simulink model "ProyectoFinal"  (R2018b)
settings: Solver=VariableStepAuto  StartTime=0.0  StopTime=100  RelTol=1e-3
libraries: simulink x3
settings Model: Creator=alvar  LastModifiedBy=alvar

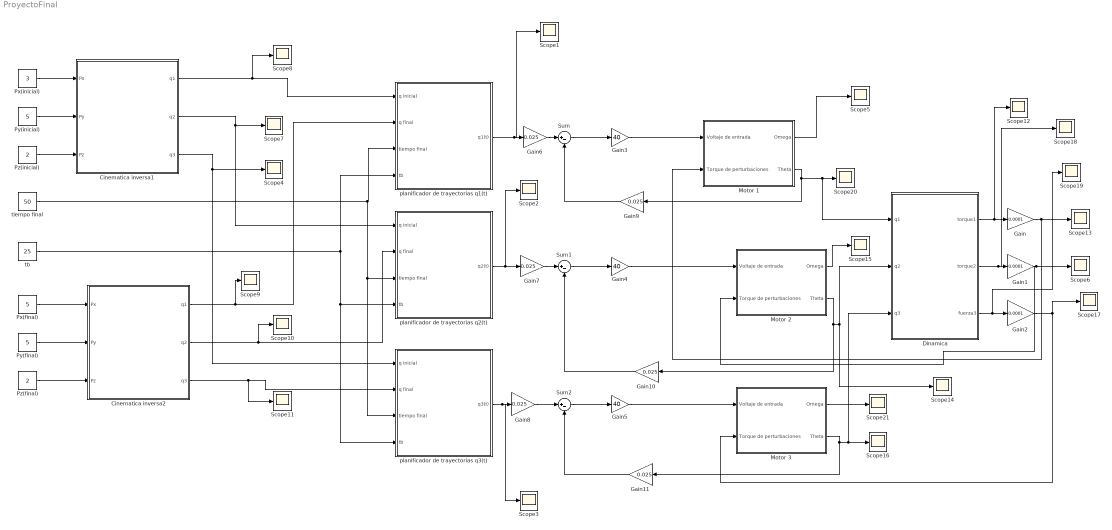
== system ProyectoFinal ==
  Cinematica inversa1 : Subsystem
  Cinematica inversa2 : Subsystem
  Dinamica : Subsystem
  Gain : Gain  Gain=0.0001
  Gain1 : Gain  Gain=0.0001
  Gain{6..11} (6 alike) : Gain  Gain=0.025
  Gain2 : Gain  Gain=0.0001
  Gain3 : Gain  Gain=40
  Gain4 : Gain  Gain=40
  Gain5 : Gain  Gain=40
  "Motor 1 " : Subsystem
  "Motor 2 " : Subsystem
  Motor 3 : Subsystem
  Px(final) : Constant  Value=5
  Px(inicial) : Constant  Value=3
  Py(final) : Constant  Value=5
  Py(inicial) : Constant  Value=5
  Pz(final) : Constant  Value=2
  Pz(inicial) : Constant  Value=2
  Scope{1..21} (21 alike) : Scope
  Sum : Sum  Inputs=|+-
  Sum1 : Sum  Inputs=|+-
  Sum2 : Sum  Inputs=|+-
  planificador de trayectorias q1(t) : Subsystem
  planificador de trayectorias q2(t) : Subsystem
  planificador de trayectorias q3(t) : Subsystem
  tb : Constant  Value=25
  tiempo final : Constant  Value=50
  wires:
  Motor 3/1(Omega) -> Scope21/1
  Gain11/1 -> Sum2/2
  Gain10/1 -> Sum1/2
  Gain9/1 -> Sum/2
  Sum/1 -> Gain3/1
  Sum2/1 -> Gain5/1
  Pz(inicial)/1 -> Cinematica inversa1/3(Pz)
  Px(inicial)/1 -> Cinematica inversa1/1(Px)
  Cinematica inversa2/1(q1) -> Scope9/1, planificador de trayectorias q1(t)/2(q final)
  Cinematica inversa1/1(q1) -> Scope8/1, planificador de trayectorias q1(t)/1(q inicial)
  Cinematica inversa1/2(q2) -> Scope7/1, planificador de trayectorias q2(t)/1(q inicial)
  Cinematica inversa2/3(q3) -> Scope11/1, planificador de trayectorias q3(t)/2(q final)
  tb/1 -> planificador de trayectorias q3(t)/4(tb), planificador de trayectorias q2(t)/4(tb), planificador de trayectorias q1(t)/4(tb)
  Gain5/1 -> Motor 3/1(Voltaje de entrada)
  Py(final)/1 -> Cinematica inversa2/2(Py)
  Py(inicial)/1 -> Cinematica inversa1/2(Py)
  Pz(final)/1 -> Cinematica inversa2/3(Pz)
  tiempo final/1 -> planificador de trayectorias q3(t)/3(tiempo final), planificador de trayectorias q2(t)/3(tiempo final), planificador de trayectorias q1(t)/3(tiempo final)
  planificador de trayectorias q2(t)/1("q2(t) ") -> Gain7/1, Scope2/1
  Px(final)/1 -> Cinematica inversa2/1(Px)
  Gain7/1 -> Sum1/1
  Gain3/1 -> "Motor 1 "/1(Voltaje de entrada)
  planificador de trayectorias q3(t)/1("q3(t) ") -> Scope3/1, Gain8/1
  Gain1/1 -> "Motor 2 "/2(Torque de perturbaciones), Scope6/1
  Dinamica/3(fuerza3) -> Scope19/1, Gain2/1
  Cinematica inversa2/2(q2) -> Scope10/1, planificador de trayectorias q2(t)/2(q final)
  planificador de trayectorias q1(t)/1("q1(t) ") -> Scope1/1, Gain6/1
  Dinamica/1(torque1) -> Scope12/1, Gain/1
  Dinamica/2(torque2) -> Scope18/1, Gain1/1
  Gain2/1 -> Motor 3/2(Torque de perturbaciones), Scope17/1
  Gain6/1 -> Sum/1
  Gain/1 -> Scope13/1, "Motor 1 "/2(Torque de perturbaciones)
  Motor 3/2(Theta) -> Gain11/1, Scope16/1, Dinamica/3(q3)
  "Motor 1 "/2(Theta) -> Dinamica/1(q1), Scope20/1, Gain9/1
  "Motor 2 "/1(Omega) -> Scope15/1
  "Motor 2 "/2(Theta) -> Scope14/1, Dinamica/2(q2), Gain10/1
  Sum1/1 -> Gain4/1
  Gain8/1 -> Sum2/1
  Cinematica inversa1/3(q3) -> Scope4/1, planificador de trayectorias q3(t)/1(q inicial)
  "Motor 1 "/1(Omega) -> Scope5/1
  Gain4/1 -> "Motor 2 "/1(Voltaje de entrada)

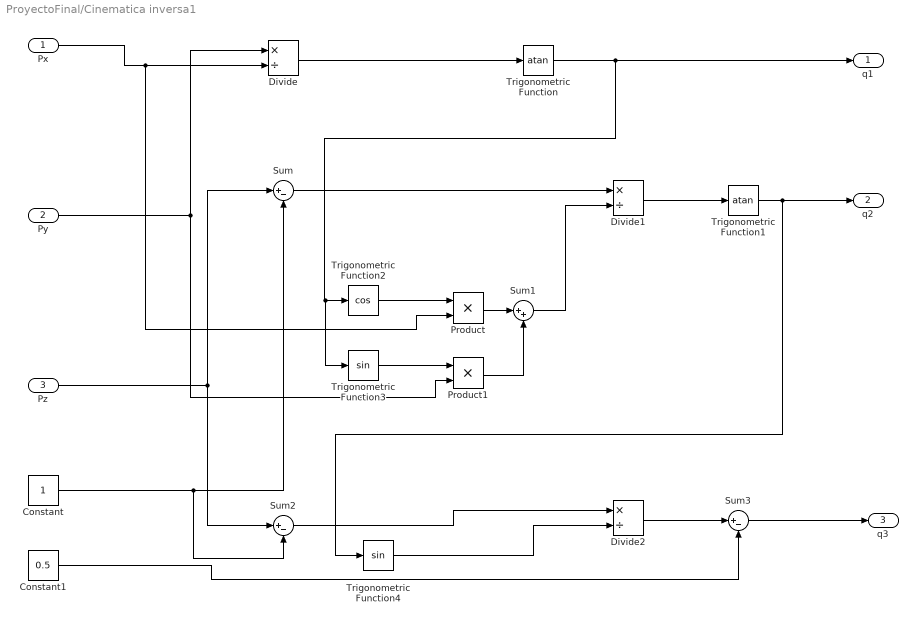
== system ProyectoFinal/Cinematica inversa1 ==
  Px : Inport
  Py : Inport  Port=2
  Pz : Inport  Port=3
  Constant : Constant
  Constant1 : Constant  Value=0.5
  Divide : Product  Inputs=*/
  Divide1 : Product  Inputs=*/
  Divide2 : Product  Inputs=*/
  Product : Product
  Product1 : Product
  Sum : Sum  Inputs=|+-
  Sum1 : Sum  Inputs=|++
  Sum2 : Sum  Inputs=|+-
  Sum3 : Sum  Inputs=|+-
  Trigonometric Function : Trigonometry  Operator=atan
  Trigonometric Function1 : Trigonometry  Operator=atan
  Trigonometric Function2 : Trigonometry  Operator=cos
  Trigonometric Function3 : Trigonometry
  Trigonometric Function4 : Trigonometry
  q1 : Outport
  q2 : Outport  Port=2
  q3 : Outport  Port=3
  wires:
  Py/1 -> Product1/2, Divide/1
  Px/1 -> Product/2, Divide/2
  Divide/1 -> Trigonometric Function/1
  Trigonometric Function/1 -> Trigonometric Function3/1, Trigonometric Function2/1, q1/1
  Pz/1 -> Sum/1, Sum2/1
  Constant/1 -> Sum2/2, Sum/2
  Sum/1 -> Divide1/1
  Trigonometric Function2/1 -> Product/1
  Product/1 -> Sum1/1
  Trigonometric Function3/1 -> Product1/1
  Product1/1 -> Sum1/2
  Sum1/1 -> Divide1/2
  Divide1/1 -> Trigonometric Function1/1
  Trigonometric Function1/1 -> Trigonometric Function4/1, q2/1
  Sum2/1 -> Divide2/1
  Trigonometric Function4/1 -> Divide2/2
  Divide2/1 -> Sum3/1
  Sum3/1 -> q3/1
  Constant1/1 -> Sum3/2

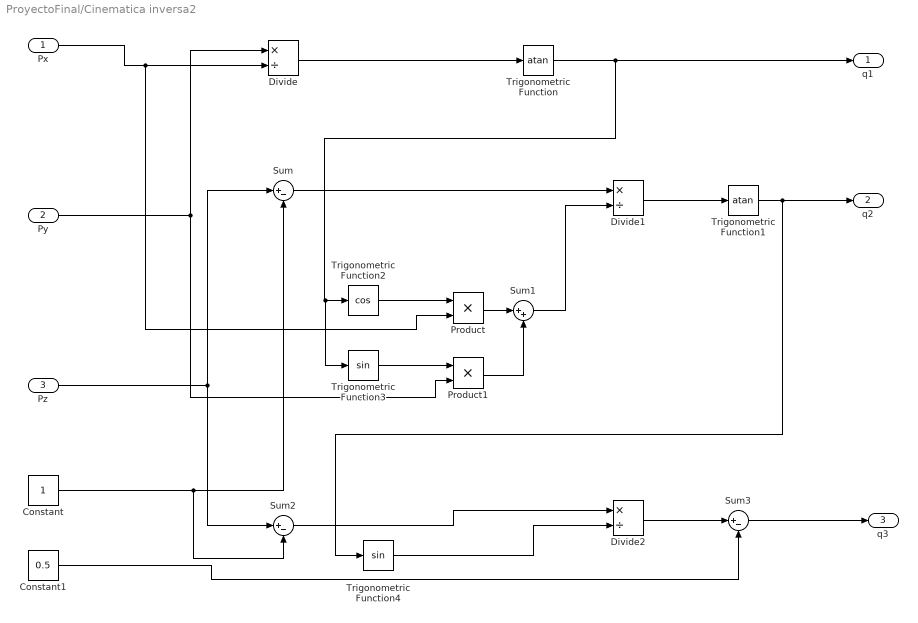
== system ProyectoFinal/Cinematica inversa2 ==
  Px : Inport
  Py : Inport  Port=2
  Pz : Inport  Port=3
  Constant : Constant
  Constant1 : Constant  Value=0.5
  Divide : Product  Inputs=*/
  Divide1 : Product  Inputs=*/
  Divide2 : Product  Inputs=*/
  Product : Product
  Product1 : Product
  Sum : Sum  Inputs=|+-
  Sum1 : Sum  Inputs=|++
  Sum2 : Sum  Inputs=|+-
  Sum3 : Sum  Inputs=|+-
  Trigonometric Function : Trigonometry  Operator=atan
  Trigonometric Function1 : Trigonometry  Operator=atan
  Trigonometric Function2 : Trigonometry  Operator=cos
  Trigonometric Function3 : Trigonometry
  Trigonometric Function4 : Trigonometry
  q1 : Outport
  q2 : Outport  Port=2
  q3 : Outport  Port=3
  wires:
  Py/1 -> Product1/2, Divide/1
  Px/1 -> Product/2, Divide/2
  Divide/1 -> Trigonometric Function/1
  Trigonometric Function/1 -> Trigonometric Function3/1, Trigonometric Function2/1, q1/1
  Pz/1 -> Sum/1, Sum2/1
  Constant/1 -> Sum2/2, Sum/2
  Sum/1 -> Divide1/1
  Trigonometric Function2/1 -> Product/1
  Product/1 -> Sum1/1
  Trigonometric Function3/1 -> Product1/1
  Product1/1 -> Sum1/2
  Sum1/1 -> Divide1/2
  Divide1/1 -> Trigonometric Function1/1
  Trigonometric Function1/1 -> Trigonometric Function4/1, q2/1
  Sum2/1 -> Divide2/1
  Trigonometric Function4/1 -> Divide2/2
  Divide2/1 -> Sum3/1
  Sum3/1 -> q3/1
  Constant1/1 -> Sum3/2

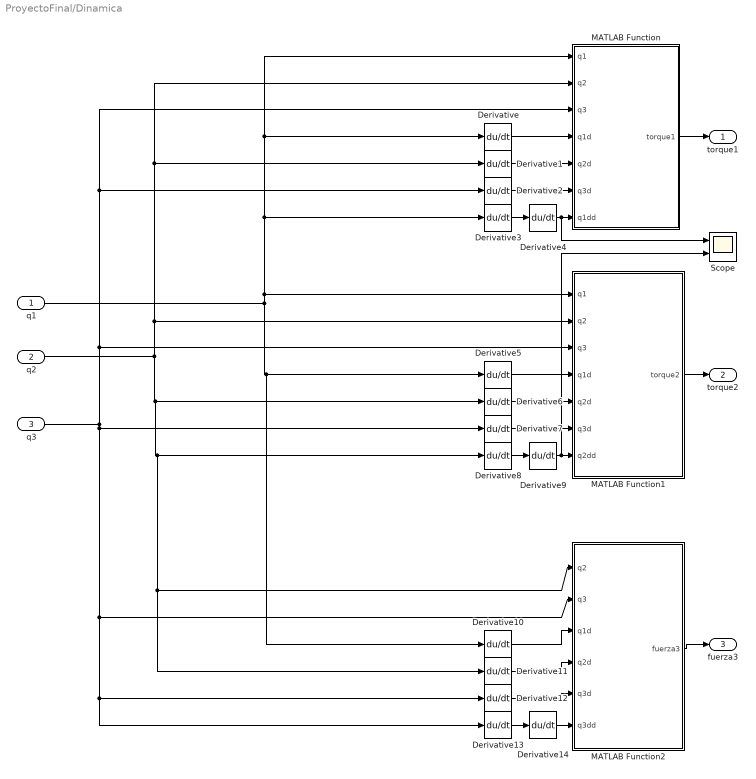
== system ProyectoFinal/Dinamica ==
  q1 : Inport
  q2 : Inport  Port=2
  q3 : Inport  Port=3
  Derivative{,1..14} (15 alike) : Derivative
  MATLAB Function : MATLAB Function  TreatAsAtomicUnit=on
  MATLAB Function1 : MATLAB Function  TreatAsAtomicUnit=on
  MATLAB Function2 : MATLAB Function  TreatAsAtomicUnit=on
  Scope : Scope  NumInputPorts=2
  torque1 : Outport
  torque2 : Outport  Port=2
  fuerza3 : Outport  Port=3
  wires:
  Derivative5/1 -> MATLAB Function1/4(q1d)
  MATLAB Function1/1(torque2) -> torque2/1
  Derivative4/1 -> Scope/1, MATLAB Function/7(q1dd)
  Derivative3/1 -> Derivative4/1
  Derivative14/1 -> MATLAB Function2/6(q3dd)
  Derivative7/1 -> MATLAB Function1/6(q3d)
  q1/1 -> Derivative10/1, Derivative5/1, MATLAB Function1/1(q1), Derivative3/1, Derivative/1, MATLAB Function/1(q1)
  Derivative6/1 -> MATLAB Function1/5(q2d)
  Derivative8/1 -> Derivative9/1
  Derivative9/1 -> Scope/2, MATLAB Function1/7(q2dd)
  Derivative1/1 -> MATLAB Function/5(q2d)
  Derivative/1 -> MATLAB Function/4(q1d)
  Derivative2/1 -> MATLAB Function/6(q3d)
  MATLAB Function2/1(fuerza3) -> fuerza3/1
  Derivative11/1 -> MATLAB Function2/4(q2d)
  Derivative13/1 -> Derivative14/1
  Derivative12/1 -> MATLAB Function2/5(q3d)
  Derivative10/1 -> MATLAB Function2/3(q1d)
  q2/1 -> MATLAB Function2/1(q2), Derivative11/1, Derivative8/1, Derivative6/1, MATLAB Function1/2(q2), Derivative1/1, MATLAB Function/2(q2)
  q3/1 -> Derivative13/1, Derivative12/1, MATLAB Function2/2(q3), Derivative7/1, MATLAB Function1/3(q3), Derivative2/1, MATLAB Function/3(q3)
  MATLAB Function/1(torque1) -> torque1/1

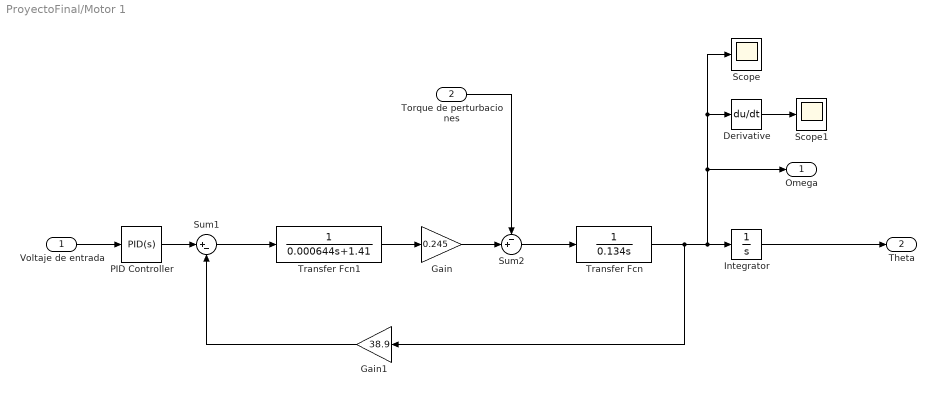
== system ProyectoFinal/Motor 1  ==
  Voltaje de entrada : Inport
  Torque de perturbaciones : Inport  Port=2
  Derivative : Derivative
  Gain : Gain  Gain=0.245
  Gain1 : Gain  Gain=38.9
  Integrator : Integrator
  PID Controller : simulink/Continuous/PID Controller  Controller=PID  Form=Parallel  TimeDomain=Continuous-time  SampleTime=-1  IntegratorMethod=Forward Euler  FilterMethod=Forward Euler  ControllerParametersSource=internal  P=12  I=4  D=5  UseFilter=on  N=100  TunerSelectOption=Transfer Function Based (PID Tuner App)  InitialConditionSource=internal  InitialConditionForIntegrator=0  InitialConditionForFilter=0  DifferentiatorICPrevScaledInput=0  ExternalReset=none  TrackingMode=off  Kt=1  LimitOutput=off  UpperSaturationLimit=inf  LowerSaturationLimit=-inf  LinearizeAsGain=on  AntiWindupMode=none  Kb=1  POutMin=[]  POutMax=[]  IOutMin=[]  IOutMax=[]  DOutMin=[]  DOutMax=[]  NOutMin=[]  NOutMax=[]  SumOutMin=[]  SumOutMax=[]  SaturationOutMin=[]  SaturationOutMax=[]  PParamMin=[]  PParamMax=[]  IParamMin=[]  IParamMax=[]  DParamMin=[]  DParamMax=[]  NParamMin=[]  NParamMax=[]  KbParamMin=[]  KbParamMax=[]  KtParamMin=[]  KtParamMax=[]  KbOutMin=[]  KbOutMax=[]  KtOutMin=[]  KtOutMax=[]  IntegratorOutMin=[]  IntegratorOutMax=[]  FilterOutMin=[]  FilterOutMax=[]  SumI1OutMin=[]  SumI1OutMax=[]  SumI2OutMin=[]  SumI2OutMax=[]  SumI3OutMin=[]  SumI3OutMax=[]  SumI4OutMin=[]  SumI4OutMax=[]  SumDOutMin=[]  SumDOutMax=[]  DifferentiatorOutMin=[]  DifferentiatorOutMax=[]  FilterDiffOutCoefMin=[]  FilterDiffOutCoefMax=[]  ReciprocalOutMin=[]  ReciprocalOutMax=[]  SumDenOutMin=[]  SumDenOutMax=[]  SumNumOutMin=[]  SumNumOutMax=[]  DivideOutMin=[]  DivideOutMax=[]  IntegratorContinuousStateAttributes=''  IntegratorStateMustResolveToSignalObject=off  IntegratorRTWStateStorageClass=Auto  FilterContinuousStateAttributes=''  FilterStateMustResolveToSignalObject=off  FilterRTWStateStorageClass=Auto  ParallelPVariant=InternalParameters  IdealPVariant=Disabled  IVariant=InternalParameters  DVariant=InternalParameters  IntegratorVariant=Continuous  SatVariant=Disabled  AWVariant=Passthrough  PCopyVariant=Disabled  TRVariant=Disabled  FdbkBlocksVariant=Forward  IdealPFdbkVariant=Disabled  SatFdbkVariant=Disabled  DerivativeFilterVariant=ContFilter  NVariant=InternalParameters  NCopyVariant=Disabled  FilterICVariant=InternalICsFilter  IntegratorICVariant=InternalICs  ExternalResetVariant=Disabled  TRSumVariant=Passthrough  SumFdbkVariant=Disabled  SumVariant=Sum_PID
  Scope : Scope
  Scope1 : Scope
  Sum1 : Sum  Inputs=|+-
  Sum2 : Sum  Inputs=-+|
  Transfer Fcn : TransferFcn  Denominator=[0.134 0]
  Transfer Fcn1 : TransferFcn  Denominator=[0.000644 1.41]
  Omega : Outport
  Theta : Outport  Port=2
  wires:
  Sum1/1 -> Transfer Fcn1/1
  Transfer Fcn1/1 -> Gain/1
  Gain1/1 -> Sum1/2
  Gain/1 -> Sum2/2
  Sum2/1 -> Transfer Fcn/1
  Torque de perturbaciones/1 -> Sum2/1
  Integrator/1 -> Theta/1
  Derivative/1 -> Scope1/1
  Transfer Fcn/1 -> Derivative/1, Scope/1, Omega/1, Integrator/1, Gain1/1
  PID Controller/1 -> Sum1/1
  Voltaje de entrada/1 -> PID Controller/1

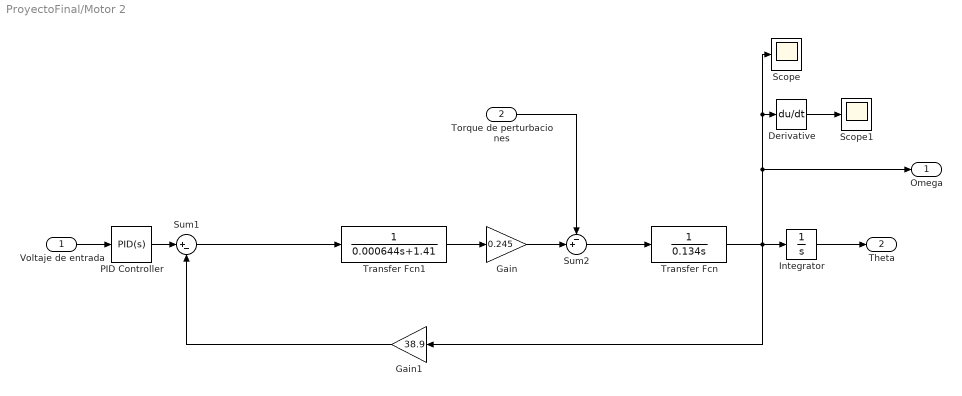
== system ProyectoFinal/Motor 2  ==
  Voltaje de entrada : Inport
  Torque de perturbaciones : Inport  Port=2
  Derivative : Derivative
  Gain : Gain  Gain=0.245
  Gain1 : Gain  Gain=38.9
  Integrator : Integrator
  PID Controller : simulink/Continuous/PID Controller  Controller=PID  Form=Parallel  TimeDomain=Continuous-time  SampleTime=-1  IntegratorMethod=Forward Euler  FilterMethod=Forward Euler  ControllerParametersSource=internal  P=12  I=4  D=5  UseFilter=on  N=100  TunerSelectOption=Transfer Function Based (PID Tuner App)  InitialConditionSource=internal  InitialConditionForIntegrator=0  InitialConditionForFilter=0  DifferentiatorICPrevScaledInput=0  ExternalReset=none  TrackingMode=off  Kt=1  LimitOutput=off  UpperSaturationLimit=inf  LowerSaturationLimit=-inf  LinearizeAsGain=on  AntiWindupMode=none  Kb=1  POutMin=[]  POutMax=[]  IOutMin=[]  IOutMax=[]  DOutMin=[]  DOutMax=[]  NOutMin=[]  NOutMax=[]  SumOutMin=[]  SumOutMax=[]  SaturationOutMin=[]  SaturationOutMax=[]  PParamMin=[]  PParamMax=[]  IParamMin=[]  IParamMax=[]  DParamMin=[]  DParamMax=[]  NParamMin=[]  NParamMax=[]  KbParamMin=[]  KbParamMax=[]  KtParamMin=[]  KtParamMax=[]  KbOutMin=[]  KbOutMax=[]  KtOutMin=[]  KtOutMax=[]  IntegratorOutMin=[]  IntegratorOutMax=[]  FilterOutMin=[]  FilterOutMax=[]  SumI1OutMin=[]  SumI1OutMax=[]  SumI2OutMin=[]  SumI2OutMax=[]  SumI3OutMin=[]  SumI3OutMax=[]  SumI4OutMin=[]  SumI4OutMax=[]  SumDOutMin=[]  SumDOutMax=[]  DifferentiatorOutMin=[]  DifferentiatorOutMax=[]  FilterDiffOutCoefMin=[]  FilterDiffOutCoefMax=[]  ReciprocalOutMin=[]  ReciprocalOutMax=[]  SumDenOutMin=[]  SumDenOutMax=[]  SumNumOutMin=[]  SumNumOutMax=[]  DivideOutMin=[]  DivideOutMax=[]  IntegratorContinuousStateAttributes=''  IntegratorStateMustResolveToSignalObject=off  IntegratorRTWStateStorageClass=Auto  FilterContinuousStateAttributes=''  FilterStateMustResolveToSignalObject=off  FilterRTWStateStorageClass=Auto  ParallelPVariant=InternalParameters  IdealPVariant=Disabled  IVariant=InternalParameters  DVariant=InternalParameters  IntegratorVariant=Continuous  SatVariant=Disabled  AWVariant=Passthrough  PCopyVariant=Disabled  TRVariant=Disabled  FdbkBlocksVariant=Forward  IdealPFdbkVariant=Disabled  SatFdbkVariant=Disabled  DerivativeFilterVariant=ContFilter  NVariant=InternalParameters  NCopyVariant=Disabled  FilterICVariant=InternalICsFilter  IntegratorICVariant=InternalICs  ExternalResetVariant=Disabled  TRSumVariant=Passthrough  SumFdbkVariant=Disabled  SumVariant=Sum_PID
  Scope : Scope
  Scope1 : Scope
  Sum1 : Sum  Inputs=|+-
  Sum2 : Sum  Inputs=-+|
  Transfer Fcn : TransferFcn  Denominator=[0.134 0]
  Transfer Fcn1 : TransferFcn  Denominator=[0.000644 1.41]
  Omega : Outport
  Theta : Outport  Port=2
  wires:
  Sum1/1 -> Transfer Fcn1/1
  Transfer Fcn1/1 -> Gain/1
  Gain1/1 -> Sum1/2
  Gain/1 -> Sum2/2
  Sum2/1 -> Transfer Fcn/1
  Torque de perturbaciones/1 -> Sum2/1
  Integrator/1 -> Theta/1
  Derivative/1 -> Scope1/1
  Transfer Fcn/1 -> Gain1/1, Omega/1, Derivative/1, Scope/1, Integrator/1
  PID Controller/1 -> Sum1/1
  Voltaje de entrada/1 -> PID Controller/1

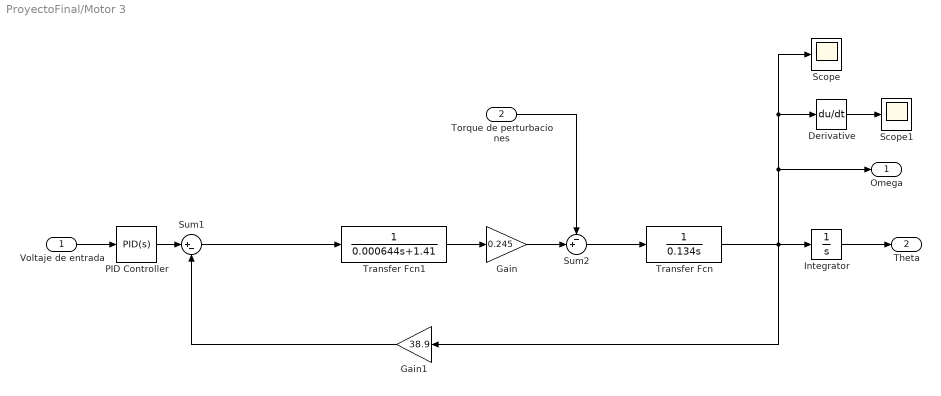
== system ProyectoFinal/Motor 3 ==
  Voltaje de entrada : Inport
  Torque de perturbaciones : Inport  Port=2
  Derivative : Derivative
  Gain : Gain  Gain=0.245
  Gain1 : Gain  Gain=38.9
  Integrator : Integrator
  PID Controller : simulink/Continuous/PID Controller  Controller=PID  Form=Parallel  TimeDomain=Continuous-time  SampleTime=-1  IntegratorMethod=Forward Euler  FilterMethod=Forward Euler  ControllerParametersSource=internal  P=12  I=4  D=5  UseFilter=on  N=100  TunerSelectOption=Transfer Function Based (PID Tuner App)  InitialConditionSource=internal  InitialConditionForIntegrator=0  InitialConditionForFilter=0  DifferentiatorICPrevScaledInput=0  ExternalReset=none  TrackingMode=off  Kt=1  LimitOutput=off  UpperSaturationLimit=inf  LowerSaturationLimit=-inf  LinearizeAsGain=on  AntiWindupMode=none  Kb=1  POutMin=[]  POutMax=[]  IOutMin=[]  IOutMax=[]  DOutMin=[]  DOutMax=[]  NOutMin=[]  NOutMax=[]  SumOutMin=[]  SumOutMax=[]  SaturationOutMin=[]  SaturationOutMax=[]  PParamMin=[]  PParamMax=[]  IParamMin=[]  IParamMax=[]  DParamMin=[]  DParamMax=[]  NParamMin=[]  NParamMax=[]  KbParamMin=[]  KbParamMax=[]  KtParamMin=[]  KtParamMax=[]  KbOutMin=[]  KbOutMax=[]  KtOutMin=[]  KtOutMax=[]  IntegratorOutMin=[]  IntegratorOutMax=[]  FilterOutMin=[]  FilterOutMax=[]  SumI1OutMin=[]  SumI1OutMax=[]  SumI2OutMin=[]  SumI2OutMax=[]  SumI3OutMin=[]  SumI3OutMax=[]  SumI4OutMin=[]  SumI4OutMax=[]  SumDOutMin=[]  SumDOutMax=[]  DifferentiatorOutMin=[]  DifferentiatorOutMax=[]  FilterDiffOutCoefMin=[]  FilterDiffOutCoefMax=[]  ReciprocalOutMin=[]  ReciprocalOutMax=[]  SumDenOutMin=[]  SumDenOutMax=[]  SumNumOutMin=[]  SumNumOutMax=[]  DivideOutMin=[]  DivideOutMax=[]  IntegratorContinuousStateAttributes=''  IntegratorStateMustResolveToSignalObject=off  IntegratorRTWStateStorageClass=Auto  FilterContinuousStateAttributes=''  FilterStateMustResolveToSignalObject=off  FilterRTWStateStorageClass=Auto  ParallelPVariant=InternalParameters  IdealPVariant=Disabled  IVariant=InternalParameters  DVariant=InternalParameters  IntegratorVariant=Continuous  SatVariant=Disabled  AWVariant=Passthrough  PCopyVariant=Disabled  TRVariant=Disabled  FdbkBlocksVariant=Forward  IdealPFdbkVariant=Disabled  SatFdbkVariant=Disabled  DerivativeFilterVariant=ContFilter  NVariant=InternalParameters  NCopyVariant=Disabled  FilterICVariant=InternalICsFilter  IntegratorICVariant=InternalICs  ExternalResetVariant=Disabled  TRSumVariant=Passthrough  SumFdbkVariant=Disabled  SumVariant=Sum_PID
  Scope : Scope
  Scope1 : Scope
  Sum1 : Sum  Inputs=|+-
  Sum2 : Sum  Inputs=-+|
  Transfer Fcn : TransferFcn  Denominator=[0.134 0]
  Transfer Fcn1 : TransferFcn  Denominator=[0.000644 1.41]
  Omega : Outport
  Theta : Outport  Port=2
  wires:
  Sum1/1 -> Transfer Fcn1/1
  Transfer Fcn1/1 -> Gain/1
  Gain1/1 -> Sum1/2
  Gain/1 -> Sum2/2
  Sum2/1 -> Transfer Fcn/1
  Torque de perturbaciones/1 -> Sum2/1
  Integrator/1 -> Theta/1
  Derivative/1 -> Scope1/1
  Transfer Fcn/1 -> Omega/1, Derivative/1, Scope/1, Integrator/1, Gain1/1
  PID Controller/1 -> Sum1/1
  Voltaje de entrada/1 -> PID Controller/1

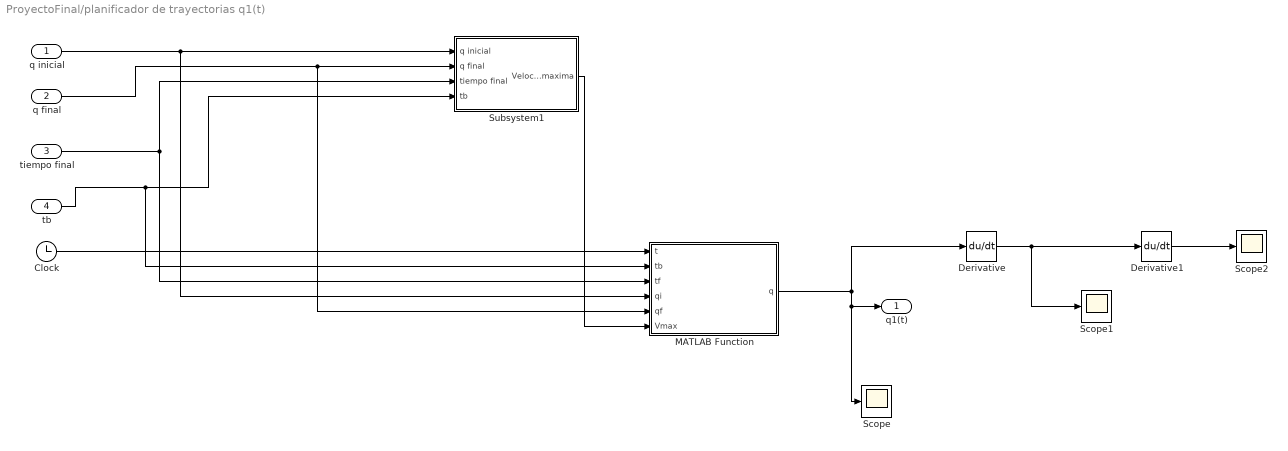
== system ProyectoFinal/planificador de trayectorias q1(t) ==
  q inicial : Inport
  q final : Inport  Port=2
  tiempo final : Inport  Port=3
  tb : Inport  Port=4
  Clock : Clock
  Derivative : Derivative
  Derivative1 : Derivative
  MATLAB Function : MATLAB Function  TreatAsAtomicUnit=on
  Scope : Scope
  Scope1 : Scope
  Scope2 : Scope
  Subsystem1 : Subsystem
  "q1(t) " : Outport
  wires:
  tb/1 -> Subsystem1/4(tb), MATLAB Function/2(tb)
  q final/1 -> MATLAB Function/5(qf), Subsystem1/2(q final)
  Derivative1/1 -> Scope2/1
  Derivative/1 -> Scope1/1, Derivative1/1
  Subsystem1/1(Velocidad maxima) -> MATLAB Function/6(Vmax)
  Clock/1 -> MATLAB Function/1(t)
  q inicial/1 -> MATLAB Function/4(qi), Subsystem1/1(q inicial)
  tiempo final/1 -> MATLAB Function/3(tf), Subsystem1/3(tiempo final)
  MATLAB Function/1(q) -> Derivative/1, "q1(t) "/1, Scope/1

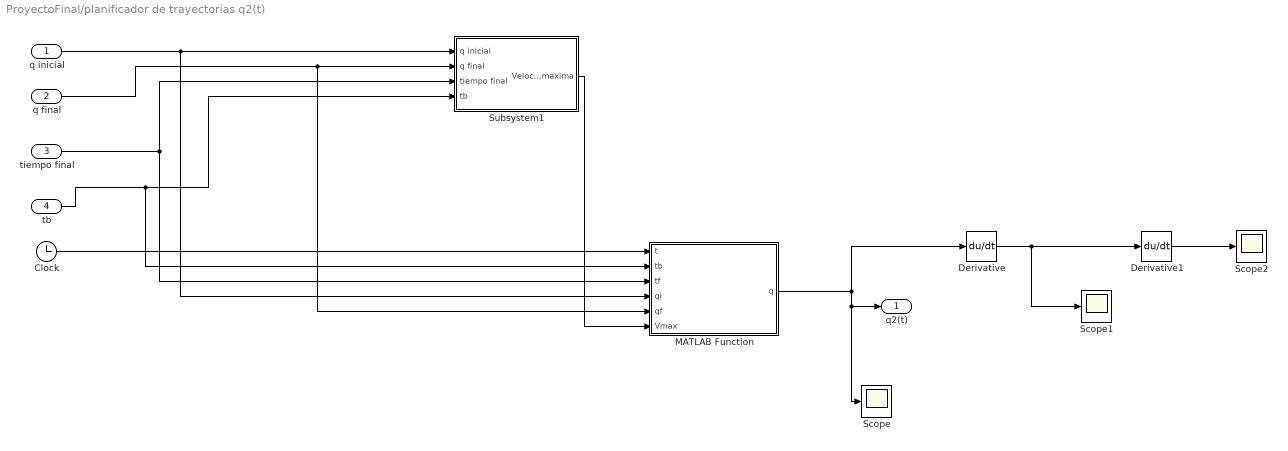
== system ProyectoFinal/planificador de trayectorias q2(t) ==
  q inicial : Inport
  q final : Inport  Port=2
  tiempo final : Inport  Port=3
  tb : Inport  Port=4
  Clock : Clock
  Derivative : Derivative
  Derivative1 : Derivative
  MATLAB Function : MATLAB Function  TreatAsAtomicUnit=on
  Scope : Scope
  Scope1 : Scope
  Scope2 : Scope
  Subsystem1 : Subsystem
  "q2(t) " : Outport
  wires:
  tb/1 -> Subsystem1/4(tb), MATLAB Function/2(tb)
  q final/1 -> MATLAB Function/5(qf), Subsystem1/2(q final)
  Derivative1/1 -> Scope2/1
  Derivative/1 -> Scope1/1, Derivative1/1
  Subsystem1/1(Velocidad maxima) -> MATLAB Function/6(Vmax)
  Clock/1 -> MATLAB Function/1(t)
  q inicial/1 -> MATLAB Function/4(qi), Subsystem1/1(q inicial)
  tiempo final/1 -> MATLAB Function/3(tf), Subsystem1/3(tiempo final)
  MATLAB Function/1(q) -> Derivative/1, "q2(t) "/1, Scope/1

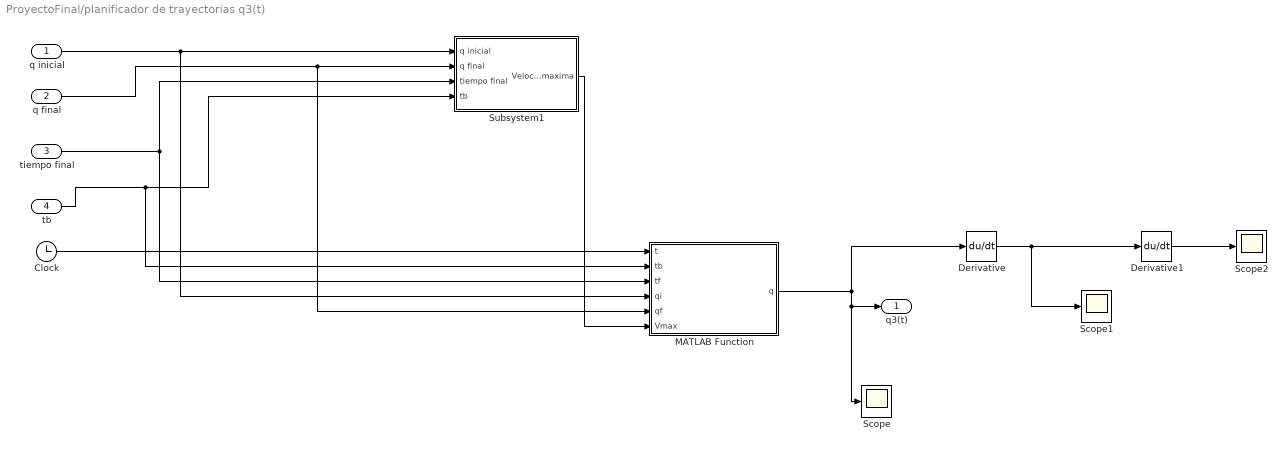
== system ProyectoFinal/planificador de trayectorias q3(t) ==
  q inicial : Inport
  q final : Inport  Port=2
  tiempo final : Inport  Port=3
  tb : Inport  Port=4
  Clock : Clock
  Derivative : Derivative
  Derivative1 : Derivative
  MATLAB Function : MATLAB Function  TreatAsAtomicUnit=on
  Scope : Scope
  Scope1 : Scope
  Scope2 : Scope
  Subsystem1 : Subsystem
  "q3(t) " : Outport
  wires:
  tb/1 -> Subsystem1/4(tb), MATLAB Function/2(tb)
  q final/1 -> MATLAB Function/5(qf), Subsystem1/2(q final)
  Derivative1/1 -> Scope2/1
  Derivative/1 -> Scope1/1, Derivative1/1
  Subsystem1/1(Velocidad maxima) -> MATLAB Function/6(Vmax)
  Clock/1 -> MATLAB Function/1(t)
  q inicial/1 -> MATLAB Function/4(qi), Subsystem1/1(q inicial)
  tiempo final/1 -> MATLAB Function/3(tf), Subsystem1/3(tiempo final)
  MATLAB Function/1(q) -> Derivative/1, "q3(t) "/1, Scope/1

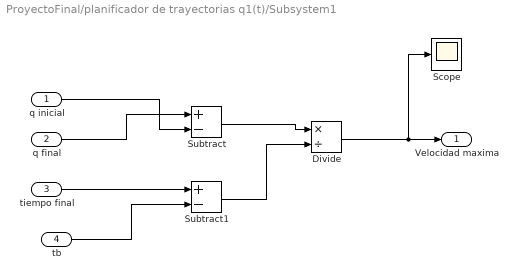
== system ProyectoFinal/planificador de trayectorias q1(t)/Subsystem1 ==
  q inicial : Inport
  q final : Inport  Port=2
  tiempo final : Inport  Port=3
  tb : Inport  Port=4
  Divide : Product  Inputs=*/
  Scope : Scope
  Subtract : Sum  Inputs=+-
  Subtract1 : Sum  Inputs=+-
  Velocidad maxima : Outport
  wires:
  q final/1 -> Subtract/1
  q inicial/1 -> Subtract/2
  Subtract/1 -> Divide/1
  Divide/1 -> Scope/1, Velocidad maxima/1
  tiempo final/1 -> Subtract1/1
  tb/1 -> Subtract1/2
  Subtract1/1 -> Divide/2

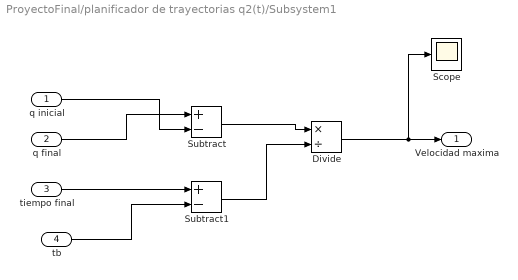
== system ProyectoFinal/planificador de trayectorias q2(t)/Subsystem1 ==
  q inicial : Inport
  q final : Inport  Port=2
  tiempo final : Inport  Port=3
  tb : Inport  Port=4
  Divide : Product  Inputs=*/
  Scope : Scope
  Subtract : Sum  Inputs=+-
  Subtract1 : Sum  Inputs=+-
  Velocidad maxima : Outport
  wires:
  q final/1 -> Subtract/1
  q inicial/1 -> Subtract/2
  Subtract/1 -> Divide/1
  Divide/1 -> Scope/1, Velocidad maxima/1
  tiempo final/1 -> Subtract1/1
  tb/1 -> Subtract1/2
  Subtract1/1 -> Divide/2

== system ProyectoFinal/planificador de trayectorias q3(t)/Subsystem1 ==
  q inicial : Inport
  q final : Inport  Port=2
  tiempo final : Inport  Port=3
  tb : Inport  Port=4
  Divide : Product  Inputs=*/
  Scope : Scope
  Subtract : Sum  Inputs=+-
  Subtract1 : Sum  Inputs=+-
  Velocidad maxima : Outport
  wires:
  q final/1 -> Subtract/1
  q inicial/1 -> Subtract/2
  Subtract/1 -> Divide/1
  Divide/1 -> Scope/1, Velocidad maxima/1
  tiempo final/1 -> Subtract1/1
  tb/1 -> Subtract1/2
  Subtract1/1 -> Divide/2

== matlab function ProyectoFinal/Dinamica/MATLAB Function1 ==
  data: q1 input; torque2 output; q2 input; q3 input; q1d input; q2d input; q3d input; q2dd input
function torque2 = fcn(q1, q2, q3, q1d, q2d, q3d, q2dd)

torque2 = q2dd*(10*(q3-0.25)^2 + 0.002 + 1*(q3+0.1)^2+0.002)+ q2d*q3d*(2*10*(q3-0.25)+2*1*(q3+0.1))+q1d^2*(-10*(q3-0.25)^2*sin(q1)*cos(q2)*q3d-sin(q2)*cos(q2)*0.002*q2d+sin(q2)*cos(q2)*q1d-1*sin(q2)*cos(q2)*0.002*q1d-1*sin(q2)*cos(q2)*(q3+0.1)^2-sin(q2)*cos(q2)*0.002*q2d+cos(q2)*sin(q2)*0.002*q2d)+10*(10*sin(q2)*(q3-0.25)+q1d+10*sin(q2)*(q3+0.1));

== matlab function ProyectoFinal/Dinamica/MATLAB Function ==
  data: q1 input; q2 input; q3 input; torque1 output; q1d input; q2d input; q3d input; q1dd input
function torque1 = fcn(q1, q2, q3, q1d, q2d, q3d, q1dd)

torque1 = q1dd*(20*(q3-0.25)^2*sin(q2)^2 + sin(q2)^2*0.002 + cos(q2)^2*0.002+ 0.008 + 1*sin(q2)^2*(q3+0.1)^2+ sin(q2)^2*0.002+ cos(q2)^2*0.002)+ q1d*q2d*(2*sin(q2)*cos(q2)*0.002-2*sin(q2)*cos(q2)+2*1*(q3+0.1)^2*sin(q2)*cos(q2)+2*10*sin(q2)*cos(q2)*(q3-0.25)^2)+q1d*q3d*(2*1*sin(q2)^2*(q3-0.25)^2+2*1*sin(q2)^2*(q3+0.1));

== matlab function ProyectoFinal/Dinamica/MATLAB Function2 ==
  data: fuerza3 output; q2 input; q3 input; q1d input; q2d input; q3d input; q3dd input
function fuerza3 = fcn(  q2, q3, q1d, q2d, q3d, q3dd)

fuerza3 = q3dd*10+ q3dd*1 - q1d^2*10*sin(q2)^2*(q3-0.25)-q2d^2*10*(q3-0.25)-q1d^2*1*sin(q2)^2*(q3+0.1)-q1d*1*(q3+0.1)-10*10*cos(q2)-10*1*cos(q2);

== matlab function ProyectoFinal/planificador de trayectorias q2(t)/MATLAB Function ==
  data: t input; q output; tb input; tf input; qi input; qf input; Vmax input
function q = fcn(t, tb, tf, qi, qf, Vmax)
q=qi;
if (t < tb)
    q = qi + Vmax*t^2/(2*tb);
elseif (t > tb) && (t < tf-tb)
    q = (qi + qf - Vmax*tf)/2 + Vmax*t;
elseif (t > tf-tb) && (t < tf)
    q = qf- Vmax*tf^2/(2*tb) + Vmax*tf*t/tb - Vmax*t^2/(2*tb);
elseif (t > tf)
    q = qf;
end

== matlab function ProyectoFinal/planificador de trayectorias q1(t)/MATLAB Function ==
  data: t input; q output; tb input; tf input; qi input; qf input; Vmax input
function q = fcn(t, tb, tf, qi, qf, Vmax)
q=qi;
if (t < tb)
    q = qi + Vmax*t^2/(2*tb);
elseif (t > tb) && (t < tf-tb)
    q = (qi + qf - Vmax*tf)/2 + Vmax*t;
elseif (t > tf-tb) && (t < tf)
    q = qf- Vmax*tf^2/(2*tb) + Vmax*tf*t/tb - Vmax*t^2/(2*tb);
elseif (t > tf)
    q = qf;
end

== matlab function ProyectoFinal/planificador de trayectorias q3(t)/MATLAB Function ==
  data: t input; q output; tb input; tf input; qi input; qf input; Vmax input
function q = fcn(t, tb, tf, qi, qf, Vmax)
q=qi;
if (t < tb)
    q = qi + Vmax*t^2/(2*tb);
elseif (t > tb) && (t < tf-tb)
    q = (qi + qf - Vmax*tf)/2 + Vmax*t;
elseif (t > tf-tb) && (t < tf)
    q = qf- Vmax*tf^2/(2*tb) + Vmax*tf*t/tb - Vmax*t^2/(2*tb);
elseif (t > tf)
    q = qf;
end
